simulink subsystem "VehicleBody1DOFLongitudinalSSC"  (R2023b)
settings: Solver=VariableStepAuto  StartTime=0.0  StopTime=10.0  RelTol=1e-3
undefined symbols (not defined in the file): EnvGrvty, PlntVehCGHgtAxl, PlntVehHtchDst, PlntVehHtchHgtAxl, PlntVehHtchLatDst, PlntWhlLdRadius
libraries: nesl_utility_internal x5, sdl_lib x1
settings Model: ModifiedByFormat=The MathWorks, Inc.  Creator=The MathWorks, Inc.  LastModifiedBy=The MathWorks, Inc.
settings OptimizationCC: ReuseModelBlockBuffer=off
settings DebuggingCC: SubsystemReferenceDiagnosticForUnitTest=warning

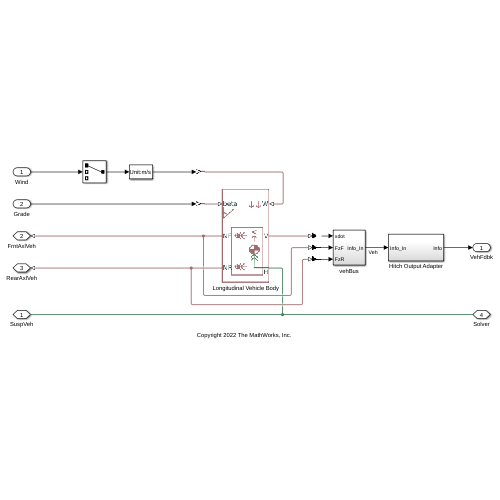
[thumbnail: Simulink's stored preview of the top-level diagram]
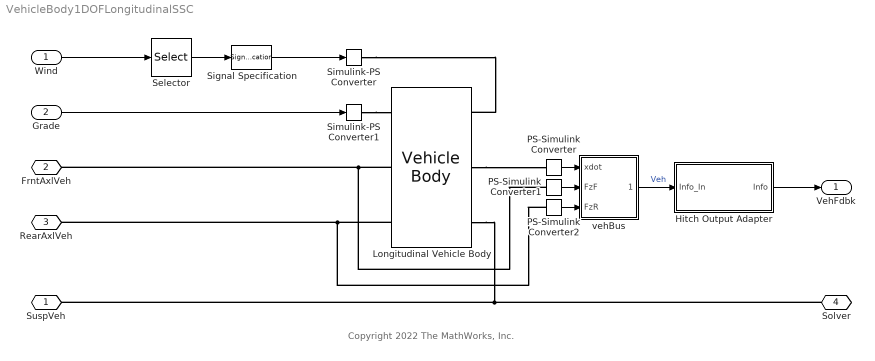
== system VehicleBody1DOFLongitudinalSSC ==
  note: Copyright 2022 The MathWorks, Inc.
  Wind : Inport  Unit=m/s
  Grade : Inport  Port=2  Unit=deg
  Hitch Output Adapter : Subsystem
  Longitudinal Vehicle Body : sdl_lib/Tires & Vehicles/Vehicle Body  mass=PlntVehMass kg  n_w=PlntVehNumWhlFrntAxl  x_f=PlntVehDstCGFrntAxl m  x_r=PlntVehDstCGRearAxl m  y_c=PlntVehCGHgtAxl+PlntWhlLdRadius m  mass_var=simscape.enum.onoff.off  g=EnvGrvty m/s^2  liftoff_warning=simscape.enum.onoff.off  area=PlntVehAeroFrntArea m^2  Cd=PlntVehAeroDragCff  rho=EnvAirDen kg/m^3  model_pitch=simscape.enum.onoff.off  inertia=4000 kg*m^2  suspension_model=sdl.enum.linearTLU.linear  k_f=1e4 N/m  b_f=1e4 N*s/m  k_r=1e4 N/m  b_r=1e4 N*s/m  k_f_TLU=[-2000, -1000, 0, 1000, 2000] N  x_f_TLU=[-.4, -.2, 0, .2, .4] m  b_f_TLU=[-200, -100, 0, 100, 200] N  v_f_TLU=[-4, -2, 0, 2, 4] m/s  k_r_TLU=[-2000, -1000, 0, 1000, 2000] N  x_r_TLU=[-.4, -.2, 0, .2, .4] m  b_r_TLU=[-200, -100, 0, 100, 200] N  v_r_TLU=[-4, -2, 0, 2, 4] m/s  interp_method=simscape.enum.interpolation.linear  extrap_method=simscape.enum.extrapolation.linear  model_hardstop=simscape.enum.onoff.off  upper_bound_f=.25 m  lower_bound_f=-.25 m  stop_k_f=1e6 N/m  stop_b_f=150 N*s/m  upper_bound_r=.25 m  lower_bound_r=-.25 m  stop_k_r=1e6 N/m  stop_b_r=150 N*s/m  initial_pitch=0 rad  initial_pitch_rate=0 rad/s  v_specify=off  v_priority=High  v=0 m/s  v_nominal_specify=off  v_nominal_unit=m/s  v_nominal_value=1
  PS-Simulink Converter : nesl_utility_internal/PS-Simulink Converter  PhysicalDomain=network_engine_domain  SubClassName=ps_output  LeftPortType=input  RightPortType=output  PseudoPeriodic=off  Frequencies=[]  VectorFormat=inherit  Unit=inherit  AffineConversion=off
  PS-Simulink Converter1 : nesl_utility_internal/PS-Simulink Converter  PhysicalDomain=network_engine_domain  SubClassName=ps_output  LeftPortType=input  RightPortType=output  PseudoPeriodic=off  Frequencies=[]  VectorFormat=inherit  Unit=inherit  AffineConversion=off
  PS-Simulink Converter2 : nesl_utility_internal/PS-Simulink Converter  PhysicalDomain=network_engine_domain  SubClassName=ps_output  LeftPortType=input  RightPortType=output  PseudoPeriodic=off  Frequencies=[]  VectorFormat=inherit  Unit=inherit  AffineConversion=off
  Selector : Selector  InputPortWidth=3  IndexOptions=Index vector (dialog)  Indices=[1]  OutputSizes=1
  Signal Specification : SignalSpecification  Unit=m/s
  Simulink-PS Converter : nesl_utility_internal/Simulink-PS Converter  PhysicalDomain=network_engine_domain  SubClassName=ps_input  LeftPortType=input  RightPortType=output  PseudoPeriodic=off  Frequencies=[]  NoiseDistribution=none  NoiseParameters=[]  Unit=m/s  AffineConversion=off  FilteringAndDerivatives=provide  SimscapeFilterOrder=1  InputFilterTimeConstant=0.001  UdotUserProvided=0
  Simulink-PS Converter1 : nesl_utility_internal/Simulink-PS Converter  PhysicalDomain=network_engine_domain  SubClassName=ps_input  LeftPortType=input  RightPortType=output  PseudoPeriodic=off  Frequencies=[]  NoiseDistribution=none  NoiseParameters=[]  Unit=deg  AffineConversion=off  FilteringAndDerivatives=provide  SimscapeFilterOrder=1  InputFilterTimeConstant=0.001  UdotUserProvided=0
  vehBus : Subsystem
  SuspVeh : PMIOPort  Side=Right
  FrntAxlVeh : PMIOPort  Port=2  Side=Right
  RearAxlVeh : PMIOPort  Port=3  Side=Right
  Solver : PMIOPort  Port=4  Side=Right
  VehFdbk : Outport  VectorParamsAs1DForOutWhenUnconnected=off
  wires:
  Wind/1 -> Selector/1
  Hitch Output Adapter/1(Info) -> VehFdbk/1
  Selector/1 -> Signal Specification/1
  Grade/1 -> Simulink-PS Converter1/1
  Signal Specification/1 -> Simulink-PS Converter/1
  PS-Simulink Converter1/1 -> vehBus/2(FzF)
  PS-Simulink Converter/1 -> vehBus/1(xdot)
  PS-Simulink Converter2/1 -> vehBus/3(FzR)
  vehBus/1(Info_In) -> Hitch Output Adapter/1(Info_In)  "Veh"
  connections:
  Longitudinal Vehicle Body/LConn1 -- Solver/RConn1 -- SuspVeh/RConn1
  Simulink-PS Converter/RConn1 -- Longitudinal Vehicle Body/LConn3
  Simulink-PS Converter1/RConn1 -- Longitudinal Vehicle Body/RConn3
  Longitudinal Vehicle Body/RConn2 -- PS-Simulink Converter1/LConn1 -- FrntAxlVeh/RConn1
  Longitudinal Vehicle Body/RConn1 -- PS-Simulink Converter2/LConn1 -- RearAxlVeh/RConn1
  Longitudinal Vehicle Body/LConn2 -- PS-Simulink Converter/LConn1

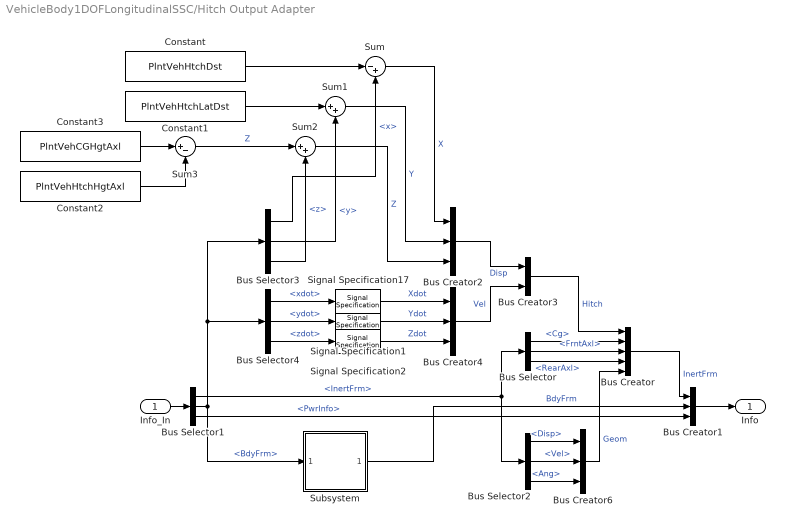
== system VehicleBody1DOFLongitudinalSSC/Hitch Output Adapter ==
  Info_In : Inport
  Bus Creator : BusCreator  Inputs=5
  Bus Creator{1..2,4,6} (4 alike) : BusCreator  Inputs=3
  Bus Creator3 : BusCreator  Inputs=2
  Bus Selector : BusSelector  OutputSignals=Cg,FrntAxl,RearAxl
  Bus Selector1 : BusSelector  OutputSignals=InertFrm,BdyFrm,PwrInfo
  Bus Selector2 : BusSelector  OutputSignals=Cg.Disp,Cg.Vel,Cg.Ang
  Bus Selector3 : BusSelector  OutputSignals=Cg.Disp.x,Cg.Disp.y,Cg.Disp.z
  Bus Selector4 : BusSelector  OutputSignals=Cg.Vel.xdot,Cg.Vel.ydot,Cg.Vel.zdot
  Constant : Constant  Value=PlntVehHtchDst  SampleTime=-1
  Constant1 : Constant  Value=PlntVehHtchLatDst  SampleTime=-1
  Constant2 : Constant  Value=PlntVehHtchHgtAxl  SampleTime=-1
  Constant3 : Constant  Value=PlntVehCGHgtAxl  SampleTime=-1
  Signal Specification1 : SignalSpecification  Unit=m/s
  Signal Specification17 : SignalSpecification  Unit=m/s
  Signal Specification2 : SignalSpecification  Unit=m/s
  Subsystem : Subsystem
  Sum : Sum  Inputs=|-+
  Sum1 : Sum  Inputs=|++
  Sum2 : Sum  Inputs=|++
  Sum3 : Sum  Inputs=|+-
  Info : Outport
  wires:
  Subsystem/1(Outport) -> Bus Creator1/2  "BdyFrm"
  Bus Selector2/3 -> Bus Creator6/3  "<Ang>"
  Bus Selector2/2 -> Bus Creator6/2  "<Vel>"
  Bus Selector2/1 -> Bus Creator6/1  "<Disp>"
  Bus Creator6/1 -> Bus Creator/5  "Geom"
  Bus Selector1/2 -> Bus Selector4/1, Bus Selector3/1, Subsystem/1(Inport)  "<BdyFrm>"
  Info_In/1 -> Bus Selector1/1
  Bus Creator/1 -> Bus Creator1/1  "InertFrm"
  Bus Selector3/3 -> Sum2/2  "<z>"
  Bus Selector/3 -> Bus Creator/4  "<RearAxl>"
  Bus Selector1/1 -> Bus Selector/1, Bus Selector2/1  "<InertFrm>"
  Bus Creator1/1 -> Info/1
  Bus Creator3/1 -> Bus Creator/1  "Hitch"
  Bus Selector1/3 -> Bus Creator1/3  "<PwrInfo>"
  Bus Selector3/1 -> Sum/2  "<x>"
  Bus Selector/1 -> Bus Creator/2  "<Cg>"
  Bus Selector/2 -> Bus Creator/3  "<FrntAxl>"
  Bus Creator4/1 -> Bus Creator3/2  "Vel"
  Bus Selector3/2 -> Sum1/2  "<y>"
  Bus Creator2/1 -> Bus Creator3/1  "Disp"
  Bus Selector4/1 -> Signal Specification17/1  "<xdot>"
  Bus Selector4/2 -> Signal Specification1/1  "<ydot>"
  Bus Selector4/3 -> Signal Specification2/1  "<zdot>"
  Constant/1 -> Sum/1
  Sum3/1 -> Sum2/1  "Z"
  Constant3/1 -> Sum3/1
  Sum2/1 -> Bus Creator2/3  "Z"
  Constant2/1 -> Sum3/2
  Sum/1 -> Bus Creator2/1  "X"
  Sum1/1 -> Bus Creator2/2  "Y"
  Constant1/1 -> Sum1/1
  Signal Specification17/1 -> Bus Creator4/1  "Xdot"
  Signal Specification1/1 -> Bus Creator4/2  "Ydot"
  Signal Specification2/1 -> Bus Creator4/3  "Zdot"

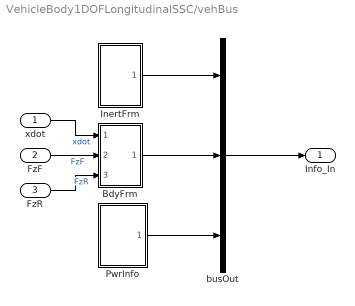
== system VehicleBody1DOFLongitudinalSSC/vehBus ==
  xdot : Inport
  FzF : Inport  Port=2
  FzR : Inport  Port=3
  BdyFrm : Subsystem
  InertFrm : Subsystem
  PwrInfo : Subsystem
  busOut : BusCreator  Inputs=3
  Info_In : Outport
  wires:
  xdot/1 -> BdyFrm/1(xdot)  "xdot"
  BdyFrm/1(BdyFrm) -> busOut/2
  InertFrm/1(InertFrm) -> busOut/1
  PwrInfo/1(PwrInfo) -> busOut/3
  busOut/1 -> Info_In/1
  FzF/1 -> BdyFrm/2(FzF)  "FzF"
  FzR/1 -> BdyFrm/3(FzR)  "FzR"

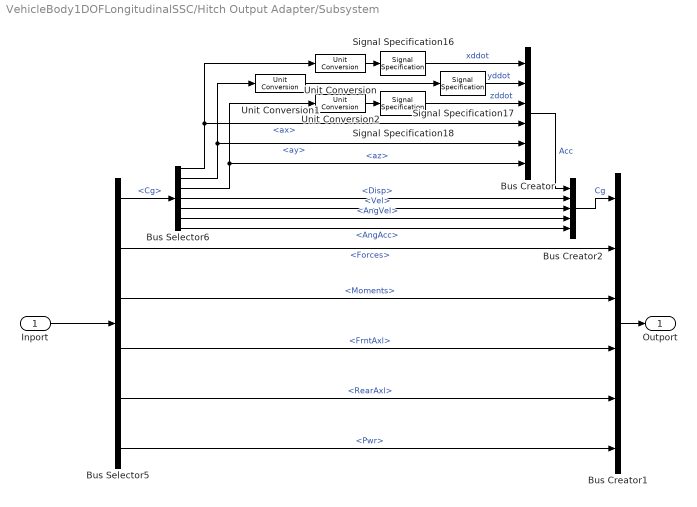
== system VehicleBody1DOFLongitudinalSSC/Hitch Output Adapter/Subsystem ==
  Inport : Inport
  Bus Creator : BusCreator  Inputs=6
  Bus Creator1 : BusCreator  Inputs=6
  Bus Creator2 : BusCreator  Inputs=5
  Bus Selector5 : BusSelector  OutputSignals=Cg,Forces,Moments,FrntAxl,RearAxl,Pwr
  Bus Selector6 : BusSelector  OutputSignals=Acc.ax,Acc.ay,Acc.az,Disp,Vel,AngVel,AngAcc
  Signal Specification16 : SignalSpecification  Unit=m/s^2
  Signal Specification17 : SignalSpecification  Unit=m/s^2
  Signal Specification18 : SignalSpecification  Unit=m/s^2
  Unit Conversion : UnitConversion
  Unit Conversion1 : UnitConversion
  Unit Conversion2 : UnitConversion
  Outport : Outport
  wires:
  Unit Conversion2/1 -> Signal Specification18/1
  Unit Conversion1/1 -> Signal Specification17/1
  Unit Conversion/1 -> Signal Specification16/1
  Bus Creator2/1 -> Bus Creator1/1  "Cg"
  Bus Selector6/6 -> Bus Creator2/4  "<AngVel>"
  Bus Selector6/7 -> Bus Creator2/5  "<AngAcc>"
  Bus Selector6/5 -> Bus Creator2/3  "<Vel>"
  Bus Selector6/4 -> Bus Creator2/2  "<Disp>"
  Bus Creator1/1 -> Outport/1
  Bus Selector5/6 -> Bus Creator1/6  "<Pwr>"
  Bus Selector5/5 -> Bus Creator1/5  "<RearAxl>"
  Bus Selector5/4 -> Bus Creator1/4  "<FrntAxl>"
  Bus Selector5/3 -> Bus Creator1/3  "<Moments>"
  Bus Selector5/2 -> Bus Creator1/2  "<Forces>"
  Bus Creator/1 -> Bus Creator2/1  "Acc"
  Bus Selector6/3 -> Bus Creator/6, Unit Conversion2/1  "<az>"
  Inport/1 -> Bus Selector5/1
  Signal Specification18/1 -> Bus Creator/3  "zddot"
  Signal Specification16/1 -> Bus Creator/1  "xddot"
  Signal Specification17/1 -> Bus Creator/2  "yddot"
  Bus Selector6/1 -> Unit Conversion/1, Bus Creator/4  "<ax>"
  Bus Selector6/2 -> Unit Conversion1/1, Bus Creator/5  "<ay>"
  Bus Selector5/1 -> Bus Selector6/1  "<Cg>"

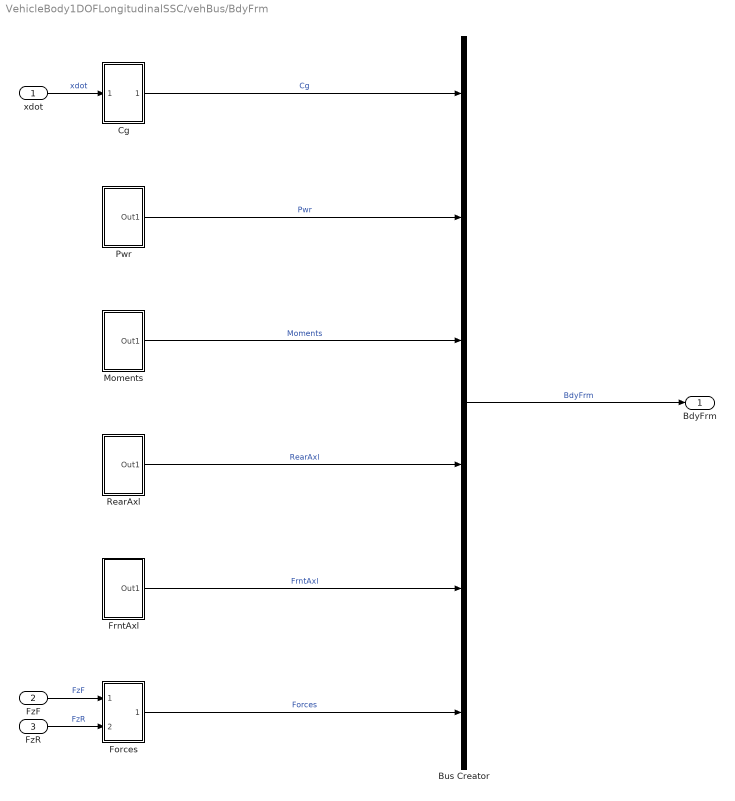
== system VehicleBody1DOFLongitudinalSSC/vehBus/BdyFrm ==
  xdot : Inport
  FzF : Inport  Port=2
  FzR : Inport  Port=3
  Bus Creator : BusCreator  Inputs=6
  Cg : Subsystem
  Forces : Subsystem
  FrntAxl : Subsystem
  Moments : Subsystem
  Pwr : Subsystem
  RearAxl : Subsystem
  BdyFrm : Outport
  wires:
  xdot/1 -> Cg/1(xdot)  "xdot"
  Cg/1(Out1) -> Bus Creator/1  "Cg"
  Forces/1(Out1) -> Bus Creator/6  "Forces"
  FrntAxl/1(Out1) -> Bus Creator/5  "FrntAxl"
  RearAxl/1(Out1) -> Bus Creator/4  "RearAxl"
  Moments/1(Out1) -> Bus Creator/3  "Moments"
  Pwr/1(Out1) -> Bus Creator/2  "Pwr"
  Bus Creator/1 -> BdyFrm/1  "BdyFrm"
  FzF/1 -> Forces/1(FzF)  "FzF"
  FzR/1 -> Forces/2(FzR)  "FzR"

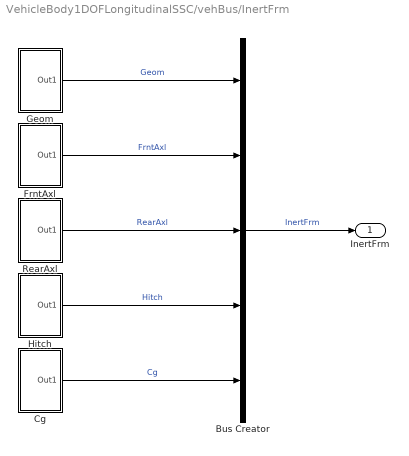
== system VehicleBody1DOFLongitudinalSSC/vehBus/InertFrm ==
  Bus Creator : BusCreator  Inputs=5
  Cg : Subsystem
  FrntAxl : Subsystem
  Geom : Subsystem
  Hitch : Subsystem
  RearAxl : Subsystem
  InertFrm : Outport
  wires:
  Hitch/1(Out1) -> Bus Creator/4  "Hitch"
  RearAxl/1(Out1) -> Bus Creator/3  "RearAxl"
  FrntAxl/1(Out1) -> Bus Creator/2  "FrntAxl"
  Geom/1(Out1) -> Bus Creator/1  "Geom"
  Cg/1(Out1) -> Bus Creator/5  "Cg"
  Bus Creator/1 -> InertFrm/1  "InertFrm"

== system VehicleBody1DOFLongitudinalSSC/vehBus/PwrInfo ==
  Bus Creator : BusCreator  Inputs=3
  vehBus_Values_PwrInfo_PwrNotTrnsfrd : Subsystem
  vehBus_Values_PwrInfo_PwrStored : Subsystem
  vehBus_Values_PwrInfo_PwrTrnsfrd : Subsystem
  PwrInfo : Outport
  wires:
  Bus Creator/1 -> PwrInfo/1  "PwrInfo"
  vehBus_Values_PwrInfo_PwrNotTrnsfrd/1(Out1) -> Bus Creator/3  "PwrNotTrnsfrd"
  vehBus_Values_PwrInfo_PwrStored/1(Out1) -> Bus Creator/2  "PwrStored"
  vehBus_Values_PwrInfo_PwrTrnsfrd/1(Out1) -> Bus Creator/1  "PwrTrnsfrd"

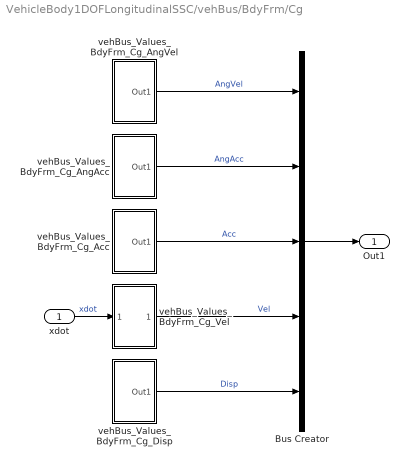
== system VehicleBody1DOFLongitudinalSSC/vehBus/BdyFrm/Cg ==
  xdot : Inport
  Bus Creator : BusCreator  Inputs=5
  vehBus_Values_BdyFrm_Cg_Acc : Subsystem
  vehBus_Values_BdyFrm_Cg_AngAcc : Subsystem
  vehBus_Values_BdyFrm_Cg_AngVel : Subsystem
  vehBus_Values_BdyFrm_Cg_Disp : Subsystem
  vehBus_Values_BdyFrm_Cg_Vel : Subsystem
  Out1 : Outport
  wires:
  xdot/1 -> vehBus_Values_BdyFrm_Cg_Vel/1(xdot)  "xdot"
  Bus Creator/1 -> Out1/1
  vehBus_Values_BdyFrm_Cg_AngAcc/1(Out1) -> Bus Creator/2  "AngAcc"
  vehBus_Values_BdyFrm_Cg_Acc/1(Out1) -> Bus Creator/3  "Acc"
  vehBus_Values_BdyFrm_Cg_AngVel/1(Out1) -> Bus Creator/1  "AngVel"
  vehBus_Values_BdyFrm_Cg_Disp/1(Out1) -> Bus Creator/5  "Disp"
  vehBus_Values_BdyFrm_Cg_Vel/1(Out1) -> Bus Creator/4  "Vel"

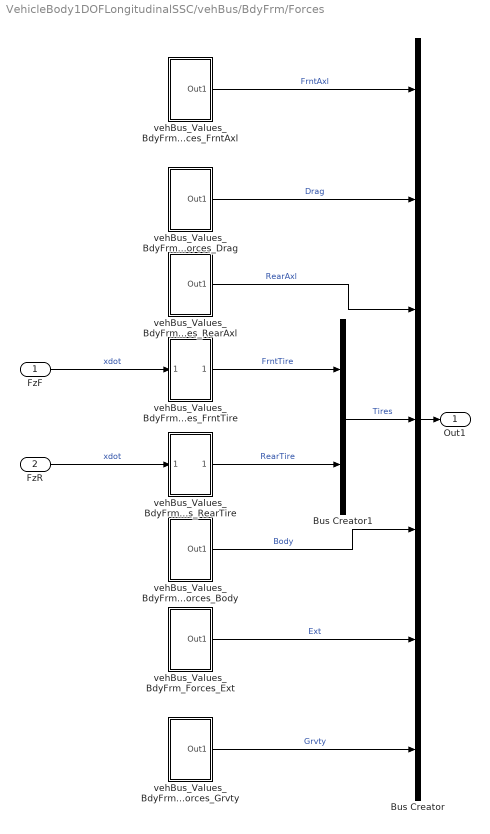
== system VehicleBody1DOFLongitudinalSSC/vehBus/BdyFrm/Forces ==
  FzF : Inport
  FzR : Inport  Port=2
  Bus Creator : BusCreator  Inputs=7
  Bus Creator1 : BusCreator  Inputs=2
  vehBus_Values_BdyFrm_Forces_Body : Subsystem
  vehBus_Values_BdyFrm_Forces_Drag : Subsystem
  vehBus_Values_BdyFrm_Forces_Ext : Subsystem
  vehBus_Values_BdyFrm_Forces_FrntAxl : Subsystem
  vehBus_Values_BdyFrm_Forces_Grvty : Subsystem
  vehBus_Values_BdyFrm_Forces_RearAxl : Subsystem
  vehBus_Values_BdyFrm_Forces_Tires_FrntTire : Subsystem
  vehBus_Values_BdyFrm_Forces_Tires_RearTire : Subsystem
  Out1 : Outport
  wires:
  Bus Creator/1 -> Out1/1
  vehBus_Values_BdyFrm_Forces_Ext/1(Out1) -> Bus Creator/6  "Ext"
  vehBus_Values_BdyFrm_Forces_RearAxl/1(Out1) -> Bus Creator/3  "RearAxl"
  vehBus_Values_BdyFrm_Forces_Tires_FrntTire/1(Out1) -> Bus Creator1/1  "FrntTire"
  vehBus_Values_BdyFrm_Forces_Body/1(Out1) -> Bus Creator/5  "Body"
  vehBus_Values_BdyFrm_Forces_Tires_RearTire/1(Out1) -> Bus Creator1/2  "RearTire"
  vehBus_Values_BdyFrm_Forces_Grvty/1(Out1) -> Bus Creator/7  "Grvty"
  vehBus_Values_BdyFrm_Forces_Drag/1(Out1) -> Bus Creator/2  "Drag"
  vehBus_Values_BdyFrm_Forces_FrntAxl/1(Out1) -> Bus Creator/1  "FrntAxl"
  FzF/1 -> vehBus_Values_BdyFrm_Forces_Tires_FrntTire/1(FzF)  "xdot"
  FzR/1 -> vehBus_Values_BdyFrm_Forces_Tires_RearTire/1(FzR)  "xdot"
  Bus Creator1/1 -> Bus Creator/4  "Tires"

== system VehicleBody1DOFLongitudinalSSC/vehBus/BdyFrm/FrntAxl ==
  Bus Creator1 : BusCreator  Inputs=3
  vehBus_Values_BdyFrm_FrntAxl_Disp : Subsystem
  vehBus_Values_BdyFrm_FrntAxl_Steer : Subsystem
  vehBus_Values_BdyFrm_FrntAxl_Vel : Subsystem
  Out1 : Outport
  wires:
  Bus Creator1/1 -> Out1/1
  vehBus_Values_BdyFrm_FrntAxl_Disp/1(Out1) -> Bus Creator1/1  "Disp"
  vehBus_Values_BdyFrm_FrntAxl_Steer/1(Out1) -> Bus Creator1/3  "Steer"
  vehBus_Values_BdyFrm_FrntAxl_Vel/1(Out1) -> Bus Creator1/2  "Vel"

== system VehicleBody1DOFLongitudinalSSC/vehBus/BdyFrm/Moments ==
  Bus Creator2 : BusCreator  Inputs=3
  vehBus_Values_BdyFrm_Moments_Body : Subsystem
  vehBus_Values_BdyFrm_Moments_Drag : Subsystem
  vehBus_Values_BdyFrm_Moments_Ext : Subsystem
  Out1 : Outport
  wires:
  Bus Creator2/1 -> Out1/1
  vehBus_Values_BdyFrm_Moments_Body/1(Out1) -> Bus Creator2/1  "Body"
  vehBus_Values_BdyFrm_Moments_Drag/1(Out1) -> Bus Creator2/2  "Drag"
  vehBus_Values_BdyFrm_Moments_Ext/1(Out1) -> Bus Creator2/3  "Ext"

== system VehicleBody1DOFLongitudinalSSC/vehBus/BdyFrm/Pwr ==
  Drag : Constant  Value=zeros([1,1])  SampleTime=-1
  PwrExt : Constant  Value=zeros([1,1])  SampleTime=-1
  Signal Specification5 : SignalSpecification  Unit=W
  busOut : BusCreator  Inputs=2
  Out1 : Outport
  wires:
  Drag/1 -> busOut/2  "Drag"
  PwrExt/1 -> busOut/1  "PwrExt"
  busOut/1 -> Signal Specification5/1
  Signal Specification5/1 -> Out1/1

== system VehicleBody1DOFLongitudinalSSC/vehBus/BdyFrm/RearAxl ==
  Bus Creator : BusCreator  Inputs=3
  vehBus_Values_BdyFrm_RearAxl_Disp : Subsystem
  vehBus_Values_BdyFrm_RearAxl_Steer : Subsystem
  vehBus_Values_BdyFrm_RearAxl_Vel : Subsystem
  Out1 : Outport
  wires:
  vehBus_Values_BdyFrm_RearAxl_Disp/1(Out1) -> Bus Creator/1  "Disp"
  vehBus_Values_BdyFrm_RearAxl_Vel/1(Out1) -> Bus Creator/2  "Vel"
  vehBus_Values_BdyFrm_RearAxl_Steer/1(Out1) -> Bus Creator/3  "Steer"
  Bus Creator/1 -> Out1/1

== system VehicleBody1DOFLongitudinalSSC/vehBus/InertFrm/Cg ==
  Bus Creator4 : BusCreator  Inputs=3
  vehBus_Values_InertFrm_Cg_Ang : Subsystem
  vehBus_Values_InertFrm_Cg_Disp : Subsystem
  vehBus_Values_InertFrm_Cg_Vel : Subsystem
  Out1 : Outport
  wires:
  Bus Creator4/1 -> Out1/1
  vehBus_Values_InertFrm_Cg_Ang/1(Out1) -> Bus Creator4/3  "Ang"
  vehBus_Values_InertFrm_Cg_Vel/1(Out1) -> Bus Creator4/2  "Vel"
  vehBus_Values_InertFrm_Cg_Disp/1(Out1) -> Bus Creator4/1  "Disp"

== system VehicleBody1DOFLongitudinalSSC/vehBus/InertFrm/FrntAxl ==
  Bus Creator : BusCreator  Inputs=2
  vehBus_Values_InertFrm_FrntAxl_Disp : Subsystem
  vehBus_Values_InertFrm_FrntAxl_Vel : Subsystem
  Out1 : Outport
  wires:
  Bus Creator/1 -> Out1/1
  vehBus_Values_InertFrm_FrntAxl_Vel/1(Out1) -> Bus Creator/2  "Vel"
  vehBus_Values_InertFrm_FrntAxl_Disp/1(Out1) -> Bus Creator/1  "Disp"

== system VehicleBody1DOFLongitudinalSSC/vehBus/InertFrm/Geom ==
  Bus Creator3 : BusCreator  Inputs=3
  vehBus_Values_InertFrm_Geom_Ang : Subsystem
  vehBus_Values_InertFrm_Geom_Disp : Subsystem
  vehBus_Values_InertFrm_Geom_Vel : Subsystem
  Out1 : Outport
  wires:
  vehBus_Values_InertFrm_Geom_Disp/1(Out1) -> Bus Creator3/1  "Disp"
  vehBus_Values_InertFrm_Geom_Ang/1(Out1) -> Bus Creator3/3  "Ang"
  vehBus_Values_InertFrm_Geom_Vel/1(Out1) -> Bus Creator3/2  "Vel"
  Bus Creator3/1 -> Out1/1

== system VehicleBody1DOFLongitudinalSSC/vehBus/InertFrm/Hitch ==
  Bus Creator2 : BusCreator  Inputs=2
  vehBus_Values_InertFrm_Hitch_Disp : Subsystem
  vehBus_Values_InertFrm_Hitch_Vel : Subsystem
  Out1 : Outport
  wires:
  Bus Creator2/1 -> Out1/1
  vehBus_Values_InertFrm_Hitch_Vel/1(Out1) -> Bus Creator2/2  "Vel"
  vehBus_Values_InertFrm_Hitch_Disp/1(Out1) -> Bus Creator2/1  "Disp"

== system VehicleBody1DOFLongitudinalSSC/vehBus/InertFrm/RearAxl ==
  Bus Creator1 : BusCreator  Inputs=2
  vehBus_Values_InertFrm_RearAxl_Disp : Subsystem
  vehBus_Values_InertFrm_RearAxl_Vel : Subsystem
  Out1 : Outport
  wires:
  Bus Creator1/1 -> Out1/1
  vehBus_Values_InertFrm_RearAxl_Vel/1(Out1) -> Bus Creator1/2  "Vel"
  vehBus_Values_InertFrm_RearAxl_Disp/1(Out1) -> Bus Creator1/1  "Disp"

== system VehicleBody1DOFLongitudinalSSC/vehBus/PwrInfo/vehBus_Values_PwrInfo_PwrNotTrnsfrd ==
  PwrFxDrag : Constant  Value=zeros([1,1])  SampleTime=-1
  Signal Specification5 : SignalSpecification  Unit=W
  busOut : BusCreator  Inputs=1
  Out1 : Outport
  wires:
  busOut/1 -> Signal Specification5/1
  PwrFxDrag/1 -> busOut/1  "PwrFxDrag"
  Signal Specification5/1 -> Out1/1

== system VehicleBody1DOFLongitudinalSSC/vehBus/PwrInfo/vehBus_Values_PwrInfo_PwrStored ==
  PwrStoredGrvty : Constant  Value=zeros([1,1])  SampleTime=-1
  PwrStoredxdot : Constant  Value=zeros([1,1])  SampleTime=-1
  Signal Specification5 : SignalSpecification  Unit=W
  busOut : BusCreator  Inputs=2
  Out1 : Outport
  wires:
  PwrStoredxdot/1 -> busOut/2  "PwrStoredxdot"
  PwrStoredGrvty/1 -> busOut/1  "PwrStoredGrvty"
  busOut/1 -> Signal Specification5/1
  Signal Specification5/1 -> Out1/1

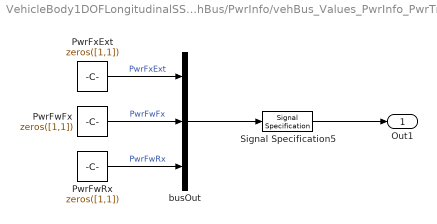
== system VehicleBody1DOFLongitudinalSSC/vehBus/PwrInfo/vehBus_Values_PwrInfo_PwrTrnsfrd ==
  PwrFwFx : Constant  Value=zeros([1,1])  SampleTime=-1
  PwrFwRx : Constant  Value=zeros([1,1])  SampleTime=-1
  PwrFxExt : Constant  Value=zeros([1,1])  SampleTime=-1
  Signal Specification5 : SignalSpecification  Unit=W
  busOut : BusCreator  Inputs=3
  Out1 : Outport
  wires:
  busOut/1 -> Signal Specification5/1
  PwrFxExt/1 -> busOut/1  "PwrFxExt"
  PwrFwFx/1 -> busOut/2  "PwrFwFx"
  PwrFwRx/1 -> busOut/3  "PwrFwRx"
  Signal Specification5/1 -> Out1/1

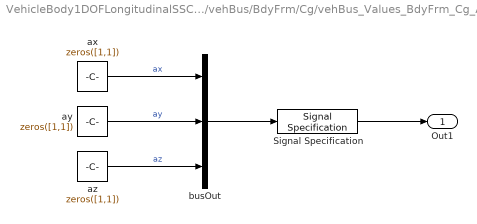
== system VehicleBody1DOFLongitudinalSSC/vehBus/BdyFrm/Cg/vehBus_Values_BdyFrm_Cg_Acc ==
  Signal Specification : SignalSpecification  Unit=m/s^2
  ax : Constant  Value=zeros([1,1])  SampleTime=-1
  ay : Constant  Value=zeros([1,1])  SampleTime=-1
  az : Constant  Value=zeros([1,1])  SampleTime=-1
  busOut : BusCreator  Inputs=3
  Out1 : Outport
  wires:
  Signal Specification/1 -> Out1/1
  busOut/1 -> Signal Specification/1
  ax/1 -> busOut/1  "ax"
  ay/1 -> busOut/2  "ay"
  az/1 -> busOut/3  "az"

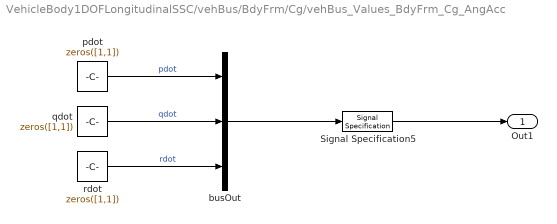
== system VehicleBody1DOFLongitudinalSSC/vehBus/BdyFrm/Cg/vehBus_Values_BdyFrm_Cg_AngAcc ==
  Signal Specification5 : SignalSpecification  Unit=rad/s^2
  busOut : BusCreator  Inputs=3
  pdot : Constant  Value=zeros([1,1])  SampleTime=-1
  qdot : Constant  Value=zeros([1,1])  SampleTime=-1
  rdot : Constant  Value=zeros([1,1])  SampleTime=-1
  Out1 : Outport
  wires:
  rdot/1 -> busOut/3  "rdot"
  busOut/1 -> Signal Specification5/1
  pdot/1 -> busOut/1  "pdot"
  qdot/1 -> busOut/2  "qdot"
  Signal Specification5/1 -> Out1/1

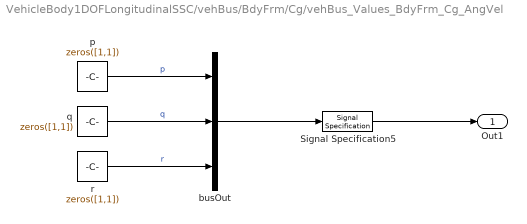
== system VehicleBody1DOFLongitudinalSSC/vehBus/BdyFrm/Cg/vehBus_Values_BdyFrm_Cg_AngVel ==
  Signal Specification5 : SignalSpecification  Unit=rad/s
  busOut : BusCreator  Inputs=3
  p : Constant  Value=zeros([1,1])  SampleTime=-1
  q : Constant  Value=zeros([1,1])  SampleTime=-1
  r : Constant  Value=zeros([1,1])  SampleTime=-1
  Out1 : Outport
  wires:
  r/1 -> busOut/3  "r"
  p/1 -> busOut/1  "p"
  busOut/1 -> Signal Specification5/1
  q/1 -> busOut/2  "q"
  Signal Specification5/1 -> Out1/1

== system VehicleBody1DOFLongitudinalSSC/vehBus/BdyFrm/Cg/vehBus_Values_BdyFrm_Cg_Disp ==
  Signal Specification5 : SignalSpecification  Unit=m
  busOut : BusCreator  Inputs=3
  x : Constant  Value=zeros([1,1])  SampleTime=-1
  y : Constant  Value=zeros([1,1])  SampleTime=-1
  z : Constant  Value=zeros([1,1])  SampleTime=-1
  Out1 : Outport
  wires:
  z/1 -> busOut/3  "z"
  y/1 -> busOut/2  "y"
  x/1 -> busOut/1  "x"
  busOut/1 -> Signal Specification5/1
  Signal Specification5/1 -> Out1/1

== system VehicleBody1DOFLongitudinalSSC/vehBus/BdyFrm/Cg/vehBus_Values_BdyFrm_Cg_Vel ==
  xdot : Inport
  Signal Specification5 : SignalSpecification  Unit=m/s
  busOut : BusCreator  Inputs=3
  ydot : Constant  Value=zeros([1,1])  SampleTime=-1
  zdot : Constant  Value=zeros([1,1])  SampleTime=-1
  Out1 : Outport
  wires:
  xdot/1 -> busOut/1  "xdot"
  zdot/1 -> busOut/3  "zdot"
  ydot/1 -> busOut/2  "ydot"
  busOut/1 -> Signal Specification5/1
  Signal Specification5/1 -> Out1/1

== system VehicleBody1DOFLongitudinalSSC/vehBus/BdyFrm/Forces/vehBus_Values_BdyFrm_Forces_Body ==
  Fx : Constant  Value=zeros([1,1])  SampleTime=-1
  Fy : Constant  Value=zeros([1,1])  SampleTime=-1
  Fz : Constant  Value=zeros([1,1])  SampleTime=-1
  Signal Specification5 : SignalSpecification  Unit=N
  busOut : BusCreator  Inputs=3
  Out1 : Outport
  wires:
  busOut/1 -> Signal Specification5/1
  Fy/1 -> busOut/2  "Fy"
  Fx/1 -> busOut/1  "Fx"
  Fz/1 -> busOut/3  "Fz"
  Signal Specification5/1 -> Out1/1

== system VehicleBody1DOFLongitudinalSSC/vehBus/BdyFrm/Forces/vehBus_Values_BdyFrm_Forces_Drag ==
  Fx : Constant  Value=zeros([1,1])  SampleTime=-1
  Fy : Constant  Value=zeros([1,1])  SampleTime=-1
  Fz : Constant  Value=zeros([1,1])  SampleTime=-1
  Signal Specification5 : SignalSpecification  Unit=N
  busOut : BusCreator  Inputs=3
  Out1 : Outport
  wires:
  Fz/1 -> busOut/3  "Fz"
  Fx/1 -> busOut/1  "Fx"
  Fy/1 -> busOut/2  "Fy"
  busOut/1 -> Signal Specification5/1
  Signal Specification5/1 -> Out1/1

== system VehicleBody1DOFLongitudinalSSC/vehBus/BdyFrm/Forces/vehBus_Values_BdyFrm_Forces_Ext ==
  Fx : Constant  Value=zeros([1,1])  SampleTime=-1
  Fy : Constant  Value=zeros([1,1])  SampleTime=-1
  Fz : Constant  Value=zeros([1,1])  SampleTime=-1
  Signal Specification5 : SignalSpecification  Unit=N
  busOut : BusCreator  Inputs=3
  Out1 : Outport
  wires:
  Fx/1 -> busOut/1  "Fx"
  busOut/1 -> Signal Specification5/1
  Fy/1 -> busOut/2  "Fy"
  Fz/1 -> busOut/3  "Fz"
  Signal Specification5/1 -> Out1/1

== system VehicleBody1DOFLongitudinalSSC/vehBus/BdyFrm/Forces/vehBus_Values_BdyFrm_Forces_FrntAxl ==
  Fx : Constant  Value=zeros([1,4526])  SampleTime=-1
  Fy : Constant  Value=zeros([1,1])  SampleTime=-1
  Fz : Constant  Value=zeros([1,1])  SampleTime=-1
  Signal Specification5 : SignalSpecification  Unit=N
  busOut : BusCreator  Inputs=3
  Out1 : Outport
  wires:
  Fz/1 -> busOut/3  "Fz"
  Fx/1 -> busOut/1  "Fx"
  busOut/1 -> Signal Specification5/1
  Fy/1 -> busOut/2  "Fy"
  Signal Specification5/1 -> Out1/1

== system VehicleBody1DOFLongitudinalSSC/vehBus/BdyFrm/Forces/vehBus_Values_BdyFrm_Forces_Grvty ==
  Fx : Constant  Value=zeros([1,1])  SampleTime=-1
  Fy : Constant  Value=zeros([1,1])  SampleTime=-1
  Fz : Constant  Value=zeros([1,1])  SampleTime=-1
  Signal Specification5 : SignalSpecification  Unit=N
  busOut : BusCreator  Inputs=3
  Out1 : Outport
  wires:
  busOut/1 -> Signal Specification5/1
  Fz/1 -> busOut/3  "Fz"
  Fy/1 -> busOut/2  "Fy"
  Fx/1 -> busOut/1  "Fx"
  Signal Specification5/1 -> Out1/1

== system VehicleBody1DOFLongitudinalSSC/vehBus/BdyFrm/Forces/vehBus_Values_BdyFrm_Forces_RearAxl ==
  Fx : Constant  Value=zeros([1,4526])  SampleTime=-1
  Fy : Constant  Value=zeros([1,1])  SampleTime=-1
  Fz : Constant  Value=zeros([1,1])  SampleTime=-1
  Signal Specification5 : SignalSpecification  Unit=N
  busOut : BusCreator  Inputs=3
  Out1 : Outport
  wires:
  busOut/1 -> Signal Specification5/1
  Fz/1 -> busOut/3  "Fz"
  Fy/1 -> busOut/2  "Fy"
  Fx/1 -> busOut/1  "Fx"
  Signal Specification5/1 -> Out1/1

== system VehicleBody1DOFLongitudinalSSC/vehBus/BdyFrm/Forces/vehBus_Values_BdyFrm_Forces_Tires_FrntTire ==
  FzF : Inport
  Fx : Constant  Value=zeros([1,1])  SampleTime=-1
  Fy : Constant  Value=zeros([1,1])  SampleTime=-1
  Signal Specification5 : SignalSpecification  Unit=N
  busOut : BusCreator  Inputs=3
  Out1 : Outport
  wires:
  busOut/1 -> Signal Specification5/1
  FzF/1 -> busOut/3  "Fz"
  Fy/1 -> busOut/2  "Fy"
  Fx/1 -> busOut/1  "Fx"
  Signal Specification5/1 -> Out1/1

== system VehicleBody1DOFLongitudinalSSC/vehBus/BdyFrm/Forces/vehBus_Values_BdyFrm_Forces_Tires_RearTire ==
  FzR : Inport
  Fx : Constant  Value=zeros([1,1])  SampleTime=-1
  Fy : Constant  Value=zeros([1,1])  SampleTime=-1
  Signal Specification5 : SignalSpecification  Unit=N
  busOut : BusCreator  Inputs=3
  Out1 : Outport
  wires:
  Fy/1 -> busOut/2  "Fy"
  FzR/1 -> busOut/3  "Fz"
  busOut/1 -> Signal Specification5/1
  Fx/1 -> busOut/1  "Fx"
  Signal Specification5/1 -> Out1/1

== system VehicleBody1DOFLongitudinalSSC/vehBus/BdyFrm/FrntAxl/vehBus_Values_BdyFrm_FrntAxl_Disp ==
  Signal Specification5 : SignalSpecification  Unit=m
  busOut : BusCreator  Inputs=3
  x : Constant  Value=zeros([1,1])  SampleTime=-1
  y : Constant  Value=zeros([1,1])  SampleTime=-1
  z : Constant  Value=zeros([1,1])  SampleTime=-1
  Out1 : Outport
  wires:
  busOut/1 -> Signal Specification5/1
  y/1 -> busOut/2  "y"
  x/1 -> busOut/1  "x"
  z/1 -> busOut/3  "z"
  Signal Specification5/1 -> Out1/1

== system VehicleBody1DOFLongitudinalSSC/vehBus/BdyFrm/FrntAxl/vehBus_Values_BdyFrm_FrntAxl_Steer ==
  Signal Specification5 : SignalSpecification  Unit=rad
  WhlAngFL : Constant  Value=zeros([1,1])  SampleTime=-1
  WhlAngFR : Constant  Value=zeros([1,1])  SampleTime=-1
  busOut : BusCreator  Inputs=2
  Out1 : Outport
  wires:
  WhlAngFL/1 -> busOut/1  "WhlAngFL"
  WhlAngFR/1 -> busOut/2  "WhlAngFR"
  busOut/1 -> Signal Specification5/1
  Signal Specification5/1 -> Out1/1

== system VehicleBody1DOFLongitudinalSSC/vehBus/BdyFrm/FrntAxl/vehBus_Values_BdyFrm_FrntAxl_Vel ==
  Signal Specification5 : SignalSpecification  Unit=m/s
  busOut : BusCreator  Inputs=3
  xdot : Constant  Value=zeros([1,1])  SampleTime=-1
  ydot : Constant  Value=zeros([1,1])  SampleTime=-1
  zdot : Constant  Value=zeros([1,1])  SampleTime=-1
  Out1 : Outport
  wires:
  busOut/1 -> Signal Specification5/1
  ydot/1 -> busOut/2  "ydot"
  xdot/1 -> busOut/1  "xdot"
  zdot/1 -> busOut/3  "zdot"
  Signal Specification5/1 -> Out1/1

== system VehicleBody1DOFLongitudinalSSC/vehBus/BdyFrm/Moments/vehBus_Values_BdyFrm_Moments_Body ==
  Mx : Constant  Value=zeros([1,1])  SampleTime=-1
  My : Constant  Value=zeros([1,1])  SampleTime=-1
  Mz : Constant  Value=zeros([1,1])  SampleTime=-1
  Signal Specification5 : SignalSpecification  Unit=N*m
  busOut : BusCreator  Inputs=3
  Out1 : Outport
  wires:
  busOut/1 -> Signal Specification5/1
  Mx/1 -> busOut/1  "Mx"
  My/1 -> busOut/2  "My"
  Mz/1 -> busOut/3  "Mz"
  Signal Specification5/1 -> Out1/1

== system VehicleBody1DOFLongitudinalSSC/vehBus/BdyFrm/Moments/vehBus_Values_BdyFrm_Moments_Drag ==
  Mx : Constant  Value=zeros([1,1])  SampleTime=-1
  My : Constant  Value=zeros([1,1])  SampleTime=-1
  Mz : Constant  Value=zeros([1,1])  SampleTime=-1
  Signal Specification5 : SignalSpecification  Unit=N*m
  busOut : BusCreator  Inputs=3
  Out1 : Outport
  wires:
  My/1 -> busOut/2  "My"
  Mz/1 -> busOut/3  "Mz"
  busOut/1 -> Signal Specification5/1
  Mx/1 -> busOut/1  "Mx"
  Signal Specification5/1 -> Out1/1

== system VehicleBody1DOFLongitudinalSSC/vehBus/BdyFrm/Moments/vehBus_Values_BdyFrm_Moments_Ext ==
  Mx : Constant  Value=zeros([1,1])  SampleTime=-1
  My : Constant  Value=zeros([1,1])  SampleTime=-1
  Mz : Constant  Value=zeros([1,1])  SampleTime=-1
  Signal Specification5 : SignalSpecification  Unit=N*m
  busOut : BusCreator  Inputs=3
  Out1 : Outport
  wires:
  busOut/1 -> Signal Specification5/1
  Mx/1 -> busOut/1  "Mx"
  My/1 -> busOut/2  "My"
  Mz/1 -> busOut/3  "Mz"
  Signal Specification5/1 -> Out1/1

== system VehicleBody1DOFLongitudinalSSC/vehBus/BdyFrm/RearAxl/vehBus_Values_BdyFrm_RearAxl_Disp ==
  Signal Specification5 : SignalSpecification  Unit=m
  busOut : BusCreator  Inputs=3
  x : Constant  Value=zeros([1,1])  SampleTime=-1
  y : Constant  Value=zeros([1,1])  SampleTime=-1
  z : Constant  Value=zeros([1,1])  SampleTime=-1
  Out1 : Outport
  wires:
  x/1 -> busOut/1  "x"
  y/1 -> busOut/2  "y"
  busOut/1 -> Signal Specification5/1
  z/1 -> busOut/3  "z"
  Signal Specification5/1 -> Out1/1

== system VehicleBody1DOFLongitudinalSSC/vehBus/BdyFrm/RearAxl/vehBus_Values_BdyFrm_RearAxl_Steer ==
  Signal Specification5 : SignalSpecification  Unit=rad
  WhlAngRL : Constant  Value=zeros([1,1])  SampleTime=-1
  WhlAngRR : Constant  Value=zeros([1,1])  SampleTime=-1
  busOut : BusCreator  Inputs=2
  Out1 : Outport
  wires:
  busOut/1 -> Signal Specification5/1
  WhlAngRL/1 -> busOut/1  "WhlAngRL"
  WhlAngRR/1 -> busOut/2  "WhlAngRR"
  Signal Specification5/1 -> Out1/1

== system VehicleBody1DOFLongitudinalSSC/vehBus/BdyFrm/RearAxl/vehBus_Values_BdyFrm_RearAxl_Vel ==
  Signal Specification5 : SignalSpecification  Unit=m/s
  busOut : BusCreator  Inputs=3
  xdot : Constant  Value=zeros([1,1])  SampleTime=-1
  ydot : Constant  Value=zeros([1,1])  SampleTime=-1
  zdot : Constant  Value=zeros([1,1])  SampleTime=-1
  Out1 : Outport
  wires:
  xdot/1 -> busOut/1  "xdot"
  zdot/1 -> busOut/3  "zdot"
  ydot/1 -> busOut/2  "ydot"
  busOut/1 -> Signal Specification5/1
  Signal Specification5/1 -> Out1/1

== system VehicleBody1DOFLongitudinalSSC/vehBus/InertFrm/Cg/vehBus_Values_InertFrm_Cg_Ang ==
  Signal Specification5 : SignalSpecification  Unit=rad
  busOut : BusCreator  Inputs=3
  phi : Constant  Value=zeros([1,1])  SampleTime=-1
  psi : Constant  Value=zeros([1,1])  SampleTime=-1
  theta : Constant  Value=zeros([1,1])  SampleTime=-1
  Out1 : Outport
  wires:
  phi/1 -> busOut/1  "phi"
  busOut/1 -> Signal Specification5/1
  theta/1 -> busOut/2  "theta"
  psi/1 -> busOut/3  "psi"
  Signal Specification5/1 -> Out1/1

== system VehicleBody1DOFLongitudinalSSC/vehBus/InertFrm/Cg/vehBus_Values_InertFrm_Cg_Disp ==
  Signal Specification5 : SignalSpecification  Unit=m
  X : Constant  Value=zeros([1,1])  SampleTime=-1
  Y : Constant  Value=zeros([1,1])  SampleTime=-1
  Z : Constant  Value=zeros([1,1])  SampleTime=-1
  busOut : BusCreator  Inputs=3
  Out1 : Outport
  wires:
  busOut/1 -> Signal Specification5/1
  Z/1 -> busOut/3  "Z"
  Y/1 -> busOut/2  "Y"
  X/1 -> busOut/1  "X"
  Signal Specification5/1 -> Out1/1

== system VehicleBody1DOFLongitudinalSSC/vehBus/InertFrm/Cg/vehBus_Values_InertFrm_Cg_Vel ==
  Signal Specification5 : SignalSpecification  Unit=m/s
  Xdot : Constant  Value=zeros([1,1])  SampleTime=-1
  Ydot : Constant  Value=zeros([1,1])  SampleTime=-1
  Zdot : Constant  Value=zeros([1,1])  SampleTime=-1
  busOut : BusCreator  Inputs=3
  Out1 : Outport
  wires:
  busOut/1 -> Signal Specification5/1
  Xdot/1 -> busOut/1  "Xdot"
  Zdot/1 -> busOut/3  "Zdot"
  Ydot/1 -> busOut/2  "Ydot"
  Signal Specification5/1 -> Out1/1

== system VehicleBody1DOFLongitudinalSSC/vehBus/InertFrm/FrntAxl/vehBus_Values_InertFrm_FrntAxl_Disp ==
  Signal Specification5 : SignalSpecification  Unit=m
  X : Constant  Value=zeros([1,1])  SampleTime=-1
  Y : Constant  Value=zeros([1,1])  SampleTime=-1
  Z : Constant  Value=zeros([1,1])  SampleTime=-1
  busOut : BusCreator  Inputs=3
  Out1 : Outport
  wires:
  X/1 -> busOut/1  "X"
  busOut/1 -> Signal Specification5/1
  Y/1 -> busOut/2  "Y"
  Z/1 -> busOut/3  "Z"
  Signal Specification5/1 -> Out1/1

== system VehicleBody1DOFLongitudinalSSC/vehBus/InertFrm/FrntAxl/vehBus_Values_InertFrm_FrntAxl_Vel ==
  Signal Specification5 : SignalSpecification  Unit=m/s
  Xdot : Constant  Value=zeros([1,1])  SampleTime=-1
  Ydot : Constant  Value=zeros([1,1])  SampleTime=-1
  Zdot : Constant  Value=zeros([1,1])  SampleTime=-1
  busOut : BusCreator  Inputs=3
  Out1 : Outport
  wires:
  busOut/1 -> Signal Specification5/1
  Ydot/1 -> busOut/2  "Ydot"
  Zdot/1 -> busOut/3  "Zdot"
  Xdot/1 -> busOut/1  "Xdot"
  Signal Specification5/1 -> Out1/1

== system VehicleBody1DOFLongitudinalSSC/vehBus/InertFrm/Geom/vehBus_Values_InertFrm_Geom_Ang ==
  Signal Specification5 : SignalSpecification  Unit=rad
  busOut : BusCreator  Inputs=3
  phi : Constant  Value=zeros([1,1])  SampleTime=-1
  psi : Constant  Value=zeros([1,1])  SampleTime=-1
  theta : Constant  Value=zeros([1,1])  SampleTime=-1
  Out1 : Outport
  wires:
  busOut/1 -> Signal Specification5/1
  phi/1 -> busOut/1  "phi"
  psi/1 -> busOut/3  "psi"
  theta/1 -> busOut/2  "theta"
  Signal Specification5/1 -> Out1/1

== system VehicleBody1DOFLongitudinalSSC/vehBus/InertFrm/Geom/vehBus_Values_InertFrm_Geom_Disp ==
  Signal Specification5 : SignalSpecification  Unit=m
  X : Constant  Value=zeros([1,1])  SampleTime=-1
  Y : Constant  Value=zeros([1,1])  SampleTime=-1
  Z : Constant  Value=zeros([1,1])  SampleTime=-1
  busOut : BusCreator  Inputs=3
  Out1 : Outport
  wires:
  busOut/1 -> Signal Specification5/1
  Z/1 -> busOut/3  "Z"
  Y/1 -> busOut/2  "Y"
  X/1 -> busOut/1  "X"
  Signal Specification5/1 -> Out1/1

== system VehicleBody1DOFLongitudinalSSC/vehBus/InertFrm/Geom/vehBus_Values_InertFrm_Geom_Vel ==
  Signal Specification5 : SignalSpecification  Unit=m/s
  Xdot : Constant  Value=zeros([1,1])  SampleTime=-1
  Ydot : Constant  Value=zeros([1,1])  SampleTime=-1
  Zdot : Constant  Value=zeros([1,1])  SampleTime=-1
  busOut : BusCreator  Inputs=3
  Out1 : Outport
  wires:
  busOut/1 -> Signal Specification5/1
  Ydot/1 -> busOut/2  "Ydot"
  Zdot/1 -> busOut/3  "Zdot"
  Xdot/1 -> busOut/1  "Xdot"
  Signal Specification5/1 -> Out1/1

== system VehicleBody1DOFLongitudinalSSC/vehBus/InertFrm/Hitch/vehBus_Values_InertFrm_Hitch_Disp ==
  Signal Specification5 : SignalSpecification  Unit=m
  X : Constant  Value=zeros([1,1])  SampleTime=-1
  Y : Constant  Value=zeros([1,1])  SampleTime=-1
  Z : Constant  Value=zeros([1,1])  SampleTime=-1
  busOut : BusCreator  Inputs=3
  Out1 : Outport
  wires:
  Z/1 -> busOut/3  "Z"
  X/1 -> busOut/1  "X"
  Y/1 -> busOut/2  "Y"
  busOut/1 -> Signal Specification5/1
  Signal Specification5/1 -> Out1/1

== system VehicleBody1DOFLongitudinalSSC/vehBus/InertFrm/Hitch/vehBus_Values_InertFrm_Hitch_Vel ==
  Signal Specification5 : SignalSpecification  Unit=m/s
  Xdot : Constant  Value=zeros([1,1])  SampleTime=-1
  Ydot : Constant  Value=zeros([1,1])  SampleTime=-1
  Zdot : Constant  Value=zeros([1,1])  SampleTime=-1
  busOut : BusCreator  Inputs=3
  Out1 : Outport
  wires:
  Xdot/1 -> busOut/1  "Xdot"
  Ydot/1 -> busOut/2  "Ydot"
  busOut/1 -> Signal Specification5/1
  Zdot/1 -> busOut/3  "Zdot"
  Signal Specification5/1 -> Out1/1

== system VehicleBody1DOFLongitudinalSSC/vehBus/InertFrm/RearAxl/vehBus_Values_InertFrm_RearAxl_Disp ==
  Signal Specification5 : SignalSpecification  Unit=m
  X : Constant  Value=zeros([1,1])  SampleTime=-1
  Y : Constant  Value=zeros([1,1])  SampleTime=-1
  Z : Constant  Value=zeros([1,1])  SampleTime=-1
  busOut : BusCreator  Inputs=3
  Out1 : Outport
  wires:
  busOut/1 -> Signal Specification5/1
  Z/1 -> busOut/3  "Z"
  X/1 -> busOut/1  "X"
  Y/1 -> busOut/2  "Y"
  Signal Specification5/1 -> Out1/1

== system VehicleBody1DOFLongitudinalSSC/vehBus/InertFrm/RearAxl/vehBus_Values_InertFrm_RearAxl_Vel ==
  Signal Specification5 : SignalSpecification  Unit=m/s
  Xdot : Constant  Value=zeros([1,1])  SampleTime=-1
  Ydot : Constant  Value=zeros([1,1])  SampleTime=-1
  Zdot : Constant  Value=zeros([1,1])  SampleTime=-1
  busOut : BusCreator  Inputs=3
  Out1 : Outport
  wires:
  busOut/1 -> Signal Specification5/1
  Ydot/1 -> busOut/2  "Ydot"
  Xdot/1 -> busOut/1  "Xdot"
  Zdot/1 -> busOut/3  "Zdot"
  Signal Specification5/1 -> Out1/1
